simulink model "ex2"  (R2019b)
settings: Solver=VariableStepAuto  StartTime=0.0  StopTime=10.0  RelTol=1e-3
libraries: slctrlblks x2, dspsrcs4 x1
settings Model: Creator=danma  LastModifiedBy=danma

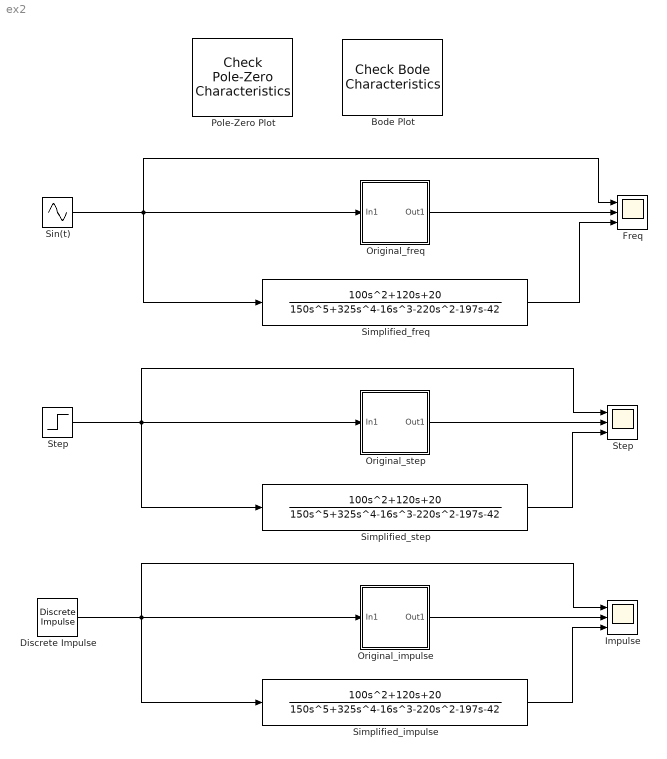
== system ex2 ==
  Bode Plot : slctrlblks/Model Verification/Check Bode  Characteristics  InstantiateOnLoad=on  SaveOperatingPoints=off  LinearizationIOs={'/Sin(t)', 1, 'in', 'off', '';'/Simplified_freq', 1, 'out', 'off', ''}  LinearizeAt=SnapshotTimes  SnapshotTimes=[0]  TriggerType=rising  SampleTime=auto  RateConversionMethod=zoh  PreWarpFreq=10  UseExactDelayModel=off  UseFullBlockNameLabels=off  UseBusSignalLabels=off  enabled=on  stopWhenAssertionFail=off  export=off  ViewDlgPos=[1 41 1920 963]  OpenViewOnLoad=off  LaunchViewOnOpen=on  FrequencyUnits=rad/s  MagnitudeUnits=dB  PhaseUnits=deg  TimeUnits=seconds  EnableUpperBound=off  UpperBoundFrequencies=[]  UpperBoundMagnitudes=[]  EnableLowerBound=off  LowerBoundFrequencies=[]  LowerBoundMagnitudes=[]
      settings: SourceProductName=Simulink Control Design
  Discrete Impulse : dspsrcs4/Discrete  Impulse  Delay=1  SampleTime=1  FrameSample=1  OutputFrames=off  dataType=double  isSigned=on  wordLen=16  udDataType=sfix(16)  fracBitsMode=Best precision  numFracBits=15  OutDataTypeStr=double  LastOutDataTypeStr=double
  Freq : Scope  NumInputPorts=3
  Impulse : Scope  NumInputPorts=3
  "Original_freq " : Subsystem
  Original_impulse : Subsystem
  Original_step : Subsystem
  Pole-Zero Plot : slctrlblks/Model Verification/Check Pole-Zero Characteristics  InstantiateOnLoad=on  SaveOperatingPoints=off  LinearizationIOs={'/Sin(t)', 1, 'in', 'off', '';'/Simplified_freq', 1, 'out', 'off', ''}  LinearizeAt=SnapshotTimes  SnapshotTimes=[0]  TriggerType=rising  SampleTime=auto  RateConversionMethod=zoh  PreWarpFreq=10  UseExactDelayModel=off  UseFullBlockNameLabels=off  UseBusSignalLabels=off  enabled=on  stopWhenAssertionFail=off  export=off  ViewDlgPos=[1 41 1920 963]  LaunchViewOnOpen=on  OpenViewOnLoad=off  FrequencyUnits=rad/s  MagnitudeUnits=dB  PhaseUnits=deg  TimeUnits=seconds  EnableSettlingTime=off  SettlingTime=[]  EnablePercentOvershoot=off  PercentOvershoot=[]  EnableDampingRatio=off  DampingRatio=[]  EnableNaturalFrequency=off  NaturalFrequencyBound=>=  NaturalFrequency=[]
      settings: SourceProductName=Simulink Control Design  SourceProductBaseCode=SD  SaveToWorkspace=off  SaveName=sys
  Simplified_freq : TransferFcn  Numerator=[100 120 20]  Denominator=[150 325 -16 -220 -197 -42]
  Simplified_impulse : TransferFcn  Numerator=[100 120 20]  Denominator=[150 325 -16 -220 -197 -42]
  Simplified_step : TransferFcn  Numerator=[100 120 20]  Denominator=[150 325 -16 -220 -197 -42]
  Sin(t) : Sin  SampleTime=0
  Step : Scope  NumInputPorts=3
  "Step " : Step  SampleTime=0
  wires:
  Sin(t)/1 -> Simplified_freq/1, Freq/1, "Original_freq "/1(In1)
  "Step "/1 -> Simplified_step/1, Step/1, Original_step/1(In1)
  "Original_freq "/1(Out1) -> Freq/2
  Simplified_freq/1 -> Freq/3
  Original_step/1(Out1) -> Step/2
  Simplified_step/1 -> Step/3
  Original_impulse/1(Out1) -> Impulse/2
  Simplified_impulse/1 -> Impulse/3
  Discrete Impulse/1 -> Impulse/1, Simplified_impulse/1, Original_impulse/1(In1)

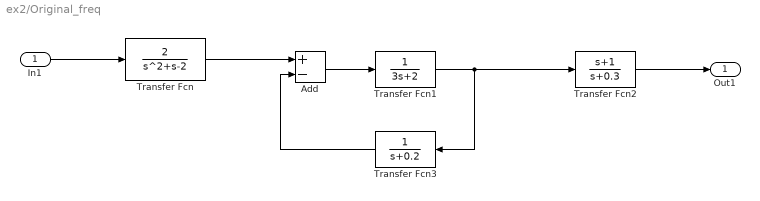
== system ex2/Original_freq  ==
  In1 : Inport
  Add : Sum  Inputs=+-
  Transfer Fcn : TransferFcn  Numerator=[2]  Denominator=[1 1 -2]
  Transfer Fcn1 : TransferFcn  Denominator=[3 2]
  Transfer Fcn2 : TransferFcn  Numerator=[1 1]  Denominator=[1 0.3]
  Transfer Fcn3 : TransferFcn  Denominator=[1 0.2]
  Out1 : Outport
  wires:
  Transfer Fcn/1 -> Add/1
  Transfer Fcn2/1 -> Out1/1
  Transfer Fcn3/1 -> Add/2
  Transfer Fcn1/1 -> Transfer Fcn3/1, Transfer Fcn2/1
  Add/1 -> Transfer Fcn1/1
  In1/1 -> Transfer Fcn/1

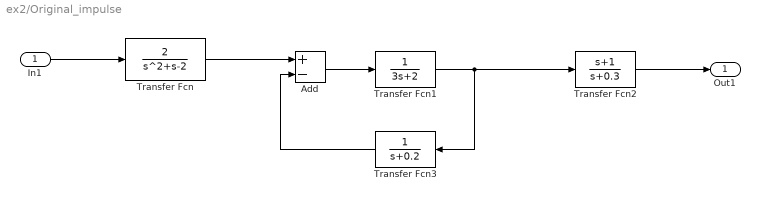
== system ex2/Original_impulse ==
  In1 : Inport
  Add : Sum  Inputs=+-
  Transfer Fcn : TransferFcn  Numerator=[2]  Denominator=[1 1 -2]
  Transfer Fcn1 : TransferFcn  Denominator=[3 2]
  Transfer Fcn2 : TransferFcn  Numerator=[1 1]  Denominator=[1 0.3]
  Transfer Fcn3 : TransferFcn  Denominator=[1 0.2]
  Out1 : Outport
  wires:
  Transfer Fcn/1 -> Add/1
  Transfer Fcn2/1 -> Out1/1
  Transfer Fcn3/1 -> Add/2
  Transfer Fcn1/1 -> Transfer Fcn3/1, Transfer Fcn2/1
  Add/1 -> Transfer Fcn1/1
  In1/1 -> Transfer Fcn/1

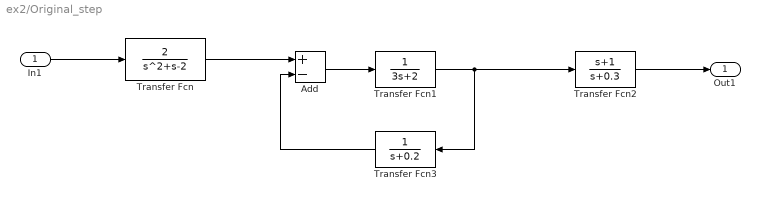
== system ex2/Original_step ==
  In1 : Inport
  Add : Sum  Inputs=+-
  Transfer Fcn : TransferFcn  Numerator=[2]  Denominator=[1 1 -2]
  Transfer Fcn1 : TransferFcn  Denominator=[3 2]
  Transfer Fcn2 : TransferFcn  Numerator=[1 1]  Denominator=[1 0.3]
  Transfer Fcn3 : TransferFcn  Denominator=[1 0.2]
  Out1 : Outport
  wires:
  Transfer Fcn/1 -> Add/1
  Transfer Fcn2/1 -> Out1/1
  Transfer Fcn3/1 -> Add/2
  Transfer Fcn1/1 -> Transfer Fcn3/1, Transfer Fcn2/1
  Add/1 -> Transfer Fcn1/1
  In1/1 -> Transfer Fcn/1
